simulink model "sl_pursuit"  (R2020a)
settings: Solver=VariableStepAuto  StartTime=0.0  StopTime=20  FixedStep=0.05  MaxStep=0.05  RelTol=1e-3  EnableMultiTasking=on
StartFcn:
  | % remove the red dashed line draw in StopFcn
  | h = findobj('Tag',  'SL_PURSUIT_PATH');
  | if ~isempty(h)
  |     delete(h)
  | end
StopFcn:
  | % get the waypoints from trajectory block
  | h = getSimulinkBlockHandle([gcs '/trajectory'])
  | path = str2num(get_param(h, 'path'));
  | 
  | % overlay it on the XY scope, tag it so it can be cleaned up in StartFcn
  | set(0, 'ShowHiddenHandles', 'on')
  | hold on
  | plot(path(:,1), path(:,2), 'Color',  'red', 'LineStyle', '--', 'LineWidth', 2, 'Tag', 'SL_PURSUIT_PATH')
  | hold off
  | set(0, 'ShowHiddenHandles', 'on')
libraries: roblocks x2, simulink x1, simulink_need_slupdate x1
settings Model: Creator=pic  LastModifiedBy=Jamie
settings DataIOCC: SaveFormat=Array  SignalLoggingSaveFormat=ModelDataLogs  TimeSaveName=t  OutputSaveName=y
settings OptimizationCC: ExpressionDepthLimit=2147483647  LifeSpan=inf
settings DebuggingCC: UnderspecifiedInitializationDetection=Classic  MergeDetectMultiDrivingBlocksExec=none  SolverPrmCheckMsg=warning  FcnCallInpInsideContextMsg=warning  AllowSymbolicDim=off  StateNameClashWarn=warning  SFUnexpectedBacktrackingDiag=warning  SFNoUnconditionalDefaultTransitionDiag=warning  SFExecutionAtInitializationDiag=none  ArithmeticOperatorsInVariantConditions=warning
settings HardwareCC: ProdBitPerPointer=32  ProdBitPerSizeT=32  ProdBitPerPtrDiffT=32  ProdLargestAtomicFloat=None  ProdIntDivRoundTo=Undefined  ProdEndianess=Unspecified  ProdWordSize=32  ProdHWDeviceType=32-bit Generic
settings ModelReferenceCC: PropagateSignalLabelsOutOfModel=off
settings SFSimCC: SimUseLocalCustomCode=off  CustomCodeUndefinedFunction=UseInterfaceOnly
settings RTWCC: RTWUseLocalCustomCode=off
settings CodeAppCC: StateflowObjectComments=on
settings GRTTargetCC: TargetLangStandard=C89/C90 (ANSI)  CombineOutputUpdateFcns=off  GRTInterface=on
settings ConfigComp: CovMetricSettings=dw  CovHtmlReporting=on  CovSaveCumulativeToWorkspaceVar=on  CovSaveSingleToWorkspaceVar=on  CovExternalEMLEnable=off

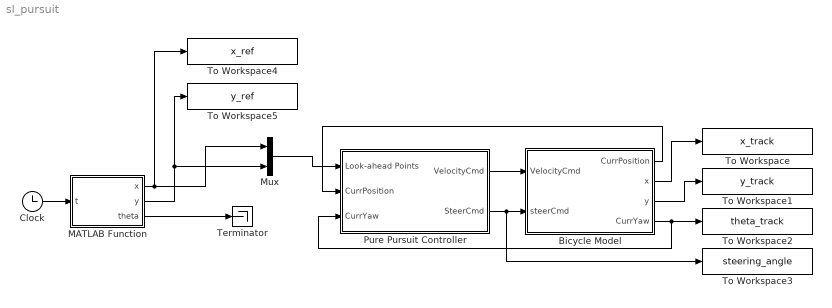
== system sl_pursuit ==
  Bicycle Model : Subsystem
  Clock : Clock
  MATLAB Function : MATLAB Function  TreatAsAtomicUnit=on
  Mux : Mux  Inputs=2
  Pure Pursuit Controller : Subsystem
  Terminator : Terminator
  To Workspace : ToWorkspace  VariableName=x_track  SampleTime=-1
      settings: Save2DSignal=2-D array (concatenate along first dimension)
  To Workspace1 : ToWorkspace  VariableName=y_track  SampleTime=-1
      settings: Save2DSignal=2-D array (concatenate along first dimension)
  To Workspace2 : ToWorkspace  VariableName=theta_track  SampleTime=-1
      settings: Save2DSignal=2-D array (concatenate along first dimension)
  To Workspace3 : ToWorkspace  VariableName=steering_angle  SampleTime=-1
      settings: Save2DSignal=2-D array (concatenate along first dimension)
  To Workspace4 : ToWorkspace  VariableName=x_ref  SampleTime=-1
      settings: Save2DSignal=2-D array (concatenate along first dimension)
  To Workspace5 : ToWorkspace  VariableName=y_ref  SampleTime=-1
      settings: Save2DSignal=2-D array (concatenate along first dimension)
  wires:
  Bicycle Model/4(CurrYaw) -> Pure Pursuit Controller/3(CurrYaw), To Workspace2/1
  Bicycle Model/2(x) -> To Workspace/1
  Bicycle Model/3(y) -> To Workspace1/1
  Pure Pursuit Controller/2(SteerCmd) -> To Workspace3/1, Bicycle Model/2(steerCmd)
  Mux/1 -> Pure Pursuit Controller/1(Look-ahead Points)
  Bicycle Model/1(CurrPosition) -> Pure Pursuit Controller/2(CurrPosition)
  Pure Pursuit Controller/1(VelocityCmd) -> Bicycle Model/1(VelocityCmd)
  MATLAB Function/1(x) -> To Workspace4/1, Mux/1
  MATLAB Function/2(y) -> Mux/2, To Workspace5/1
  MATLAB Function/3(theta) -> Terminator/1
  Clock/1 -> MATLAB Function/1(t)

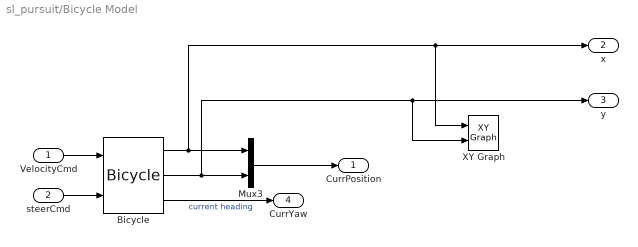
== system sl_pursuit/Bicycle Model ==
  VelocityCmd : Inport
  steerCmd : Inport  Port=2
  Bicycle : roblocks/Vehicles/Bicycle  vlim=5  accel=1  alim=0.4  steer_rate=Inf  L=0.324  x0=[0, 0, 1.57]
      link override acceleration limit: RisingSlewLimit=3  FallingSlewLimit=-3
      link override steering angle limit: UpperLimit=3  LowerLimit=-3
      link override steering rate limit: RisingSlewLimit=3  FallingSlewLimit=-3
      link override vel limit: UpperLimit=3  LowerLimit=-3
  Mux3 : Mux  Inputs=2
  XY Graph : simulink/Sinks/XY Graph  xmin=-1  xmax=4  ymin=-3  ymax=3  st=-1
  CurrPosition : Outport
  x : Outport  Port=2
  y : Outport  Port=3
  CurrYaw : Outport  Port=4
  wires:
  Mux3/1 -> CurrPosition/1
  Bicycle/1 -> XY Graph/1, x/1, Mux3/1
  steerCmd/1 -> Bicycle/2
  VelocityCmd/1 -> Bicycle/1
  Bicycle/2 -> XY Graph/2, y/1, Mux3/2
  Bicycle/3 -> CurrYaw/1  "current heading"

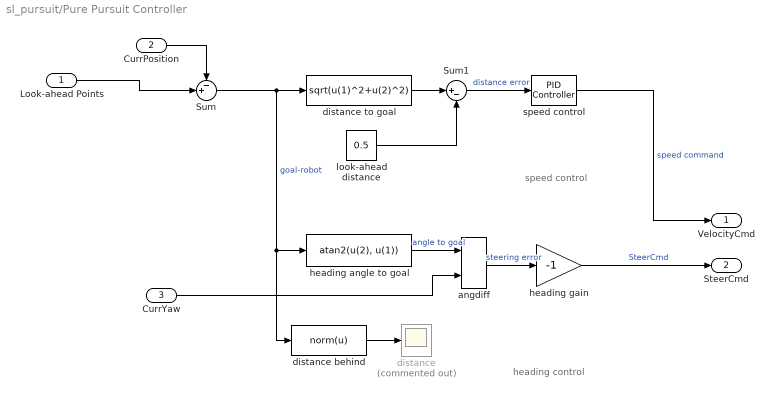
== system sl_pursuit/Pure Pursuit Controller ==
  note: speed control
  note: heading control
  Look-ahead Points : Inport
  CurrPosition : Inport  Port=2
  CurrYaw : Inport  Port=3
  Sum : Sum  Inputs=-+|
  Sum1 : Sum  Inputs=|+-
  angdiff : roblocks/Toolbox/angdiff
  distance : Scope  Commented=on
  distance behind : MATLABFcn  MATLABFcn=norm(u)
  distance to goal : Fcn  Expr=sqrt(u(1)^2+u(2)^2)
  heading angle to goal : Fcn  Expr=atan2(u(2), u(1))
  heading gain : Gain  Gain=-1
  look-ahead distance : Constant  Value=0.5
  speed control : simulink_need_slupdate/PID Controller  P=1.88  I=3  D=0.21
  VelocityCmd : Outport
  SteerCmd : Outport  Port=2
  wires:
  CurrPosition/1 -> Sum/1
  heading angle to goal/1 -> angdiff/1  "angle to goal"
  Sum/1 -> distance behind/1, heading angle to goal/1, distance to goal/1  "goal-robot"
  distance to goal/1 -> Sum1/1
  speed control/1 -> VelocityCmd/1  "speed command"
  Sum1/1 -> speed control/1  "distance error"
  angdiff/1 -> heading gain/1  "steering error"
  look-ahead distance/1 -> Sum1/2
  distance behind/1 -> distance/1
  CurrYaw/1 -> angdiff/2
  heading gain/1 -> SteerCmd/1  "SteerCmd"
  Look-ahead Points/1 -> Sum/2

== matlab function sl_pursuit/MATLAB Function ==
  data: t input; x output; y output; theta output
function [x,y,theta]= fcn(t)
pi = 3.14159;

v = 1;
R = 1;
T0 = pi*R/v;

if ((t >= 0)&&(t <= T0))
    x = R - R*cos((v/R)*t);
    y = R*sin((v/R)*t);
    theta = pi/2 - (v/R)*t;
elseif ((t >= T0)&&(t <= 3*T0))
    x = 3*R - R*cos((v/R)*(-t + T0));
    y = R*sin((v/R)*(-t + T0));
    theta = -pi/2 + (v/R)*(t - T0);
elseif ((t > 3*T0)&&(t < 4*T0))
    x = R + R*cos((v/R)*(t - 3*T0));
    y = -R*sin((v/R)*(t - 3*T0));
    theta = 3*pi/2 + (v/R)*(-t + 3*T0);
else
    x = 0;
    y = 0;
    theta = pi/2;
end
end
